simulink model "habeeb"  (R2018a)
settings: Solver=VariableStepAuto  StartTime=0.0  StopTime=100.0  RelTol=1e-3
libraries: simulink x1
settings Model: Creator=BORI  LastModifiedBy=BORI

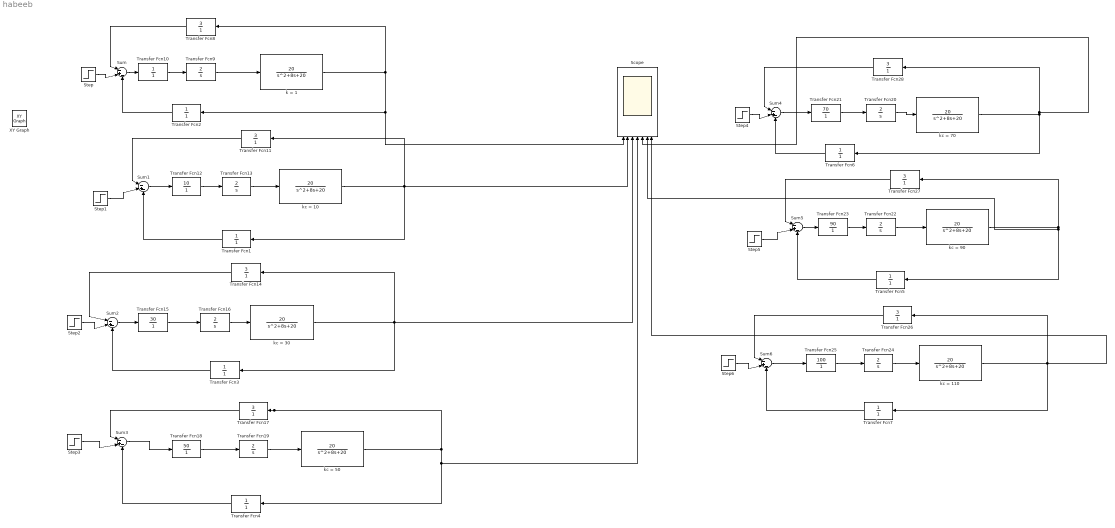
== system habeeb ==
  Scope : Scope  NumInputPorts=7
  Step{,1..6} (7 alike) : Step  SampleTime=0
  Sum{,1..6} (7 alike) : Sum  Inputs=|-+-
  Transfer Fcn{1..7,10} (8 alike) : TransferFcn  Denominator=[1]
  Transfer Fcn{8,11,14,17,26..28} (7 alike) : TransferFcn  Numerator=[3]  Denominator=[1]
  Transfer Fcn12 : TransferFcn  Numerator=[10]  Denominator=[1]
  Transfer Fcn{9,13,16,19..20,22,24} (7 alike) : TransferFcn  Numerator=[2]  Denominator=[1 0]
  Transfer Fcn15 : TransferFcn  Numerator=[30]  Denominator=[1]
  Transfer Fcn18 : TransferFcn  Numerator=[50]  Denominator=[1]
  Transfer Fcn21 : TransferFcn  Numerator=[70]  Denominator=[1]
  Transfer Fcn23 : TransferFcn  Numerator=[90]  Denominator=[1]
  Transfer Fcn25 : TransferFcn  Numerator=[100]  Denominator=[1]
  k = 1 : TransferFcn  Numerator=[20]  Denominator=[1 8 20]
  kc = {10,30,50,70,90,110} (6 alike) : TransferFcn  Numerator=[20]  Denominator=[1 8 20]
  XY Graph : simulink/Sinks/XY Graph  IOType=viewer  xmin=-1  xmax=1  ymin=-1  ymax=1  st=-1
  wires:
  Sum/1 -> Transfer Fcn10/1
  k = 1/1 -> Scope/1, Transfer Fcn2/1, Transfer Fcn8/1
  Step/1 -> Sum/2
  Transfer Fcn2/1 -> Sum/3
  Transfer Fcn10/1 -> Transfer Fcn9/1
  Transfer Fcn8/1 -> Sum/1
  Transfer Fcn11/1 -> Sum1/1
  Transfer Fcn1/1 -> Sum1/3
  Step1/1 -> Sum1/2
  Sum1/1 -> Transfer Fcn12/1
  kc = 10/1 -> Transfer Fcn11/1, Transfer Fcn1/1, Scope/2
  kc = 30/1 -> Transfer Fcn14/1, Transfer Fcn3/1, Scope/3
  Transfer Fcn3/1 -> Sum2/3
  Step2/1 -> Sum2/2
  kc = 50/1 -> Scope/4, Transfer Fcn4/1, Transfer Fcn17/1
  Transfer Fcn17/1 -> Sum3/1
  Transfer Fcn4/1 -> Sum3/3
  Step3/1 -> Sum3/2
  Step4/1 -> Sum4/2
  Transfer Fcn6/1 -> Sum4/3
  Transfer Fcn28/1 -> Sum4/1
  Step5/1 -> Sum5/2
  Step6/1 -> Sum6/2
  Transfer Fcn5/1 -> Sum5/3
  Transfer Fcn7/1 -> Sum6/3
  Transfer Fcn9/1 -> k = 1/1
  Transfer Fcn12/1 -> Transfer Fcn13/1
  Transfer Fcn13/1 -> kc = 10/1
  Transfer Fcn16/1 -> kc = 30/1
  Transfer Fcn15/1 -> Transfer Fcn16/1
  Transfer Fcn19/1 -> kc = 50/1
  Transfer Fcn18/1 -> Transfer Fcn19/1
  Sum3/1 -> Transfer Fcn18/1
  Transfer Fcn21/1 -> Transfer Fcn20/1
  Sum4/1 -> Transfer Fcn21/1
  Sum5/1 -> Transfer Fcn23/1
  Transfer Fcn23/1 -> Transfer Fcn22/1
  Transfer Fcn22/1 -> kc = 90/1
  Sum6/1 -> Transfer Fcn25/1
  Transfer Fcn26/1 -> Sum6/1
  kc = 110/1 -> Transfer Fcn26/1, Scope/7, Transfer Fcn7/1
  kc = 90/1 -> Transfer Fcn27/1, Scope/6, Transfer Fcn5/1
  Transfer Fcn27/1 -> Sum5/1
  Transfer Fcn20/1 -> kc = 70/1
  Transfer Fcn14/1 -> Sum2/1
  kc = 70/1 -> Scope/5, Transfer Fcn28/1, Transfer Fcn6/1
  Sum2/1 -> Transfer Fcn15/1
  Transfer Fcn25/1 -> Transfer Fcn24/1
  Transfer Fcn24/1 -> kc = 110/1
